simulink model "simulation1_eeef366_5"  (R2017a)
settings: Solver=ode1  StartTime=0.0  StopTime=24*3600  FixedStep=60  MaxStep=60  RelTol=1e-3  EnableMultiTasking=on
InitFcn:
  | clc
  | tic
  | disp('----------------------------------')
  | disp(' ### Solving...')
  | disp('----------------------------------')
StartFcn:
  | disp(['Initialization took: ', num2str(toc), ' s'])
  | disp('Solving...')
  | tic
StopFcn:
  | dt = str2double(get_param([gcs, '/', 'powergui'], 'SampleTime'));
  | 
  | tend = str2double(get_param(gcs, 'StopTime'));
  | 
  | runTime = toc;
  | disp('----------------------------------')
  | disp(['### Simulation took: ', num2str(runTime), ' secs'])
  | 
  | disp(['### Simulation took: ', num2str(runTime/60), ' mins'])
  | 
  | numSteps = tend / dt;
  | 
  | disp(['### Steps / sec = ', num2str(numSteps / runTime)])
  | 
  | disp(['### Secs / step = ', num2str(runTime / numSteps)])
  | 
  | disp(['### Num. steps = ', num2str(numSteps)])
  | disp('----------------------------------')
libraries: powerlib x60, powerlib_extras x12, powerlib_meascontrol x1
(part 1 of 2)
settings Model: Creator=fmu57  LastModifiedBy=Aryan Ritwajeet Jha
settings DataIOCC: LimitDataPoints=on  SaveFormat=Array  SignalLoggingSaveFormat=ModelDataLogs
settings OptimizationCC: ExpressionDepthLimit=2147483647  LifeSpan=inf
settings DebuggingCC: UnderspecifiedInitializationDetection=Classic  MergeDetectMultiDrivingBlocksExec=none  SolverPrmCheckMsg=warning  StateNameClashWarn=warning  SFUnexpectedBacktrackingDiag=warning  SFNoUnconditionalDefaultTransitionDiag=warning  SFExecutionAtInitializationDiag=none
settings HardwareCC: ProdBitPerPointer=32  ProdBitPerSizeT=32  ProdBitPerPtrDiffT=32  ProdLargestAtomicFloat=None  ProdIntDivRoundTo=Undefined  ProdEndianess=Unspecified  ProdWordSize=32  ProdHWDeviceType=32-bit Generic
settings ModelReferenceCC: PropagateSignalLabelsOutOfModel=off
settings GRTTargetCC: TargetLangStandard=C89/C90 (ANSI)  GeneratePreprocessorConditionals=Disable all  CombineOutputUpdateFcns=off  GRTInterface=on
settings ConfigComp: CovMetricSettings=dw  CovHtmlReporting=on  CovSaveCumulativeToWorkspaceVar=on  CovSaveSingleToWorkspaceVar=on  CovExternalEMLEnable=off

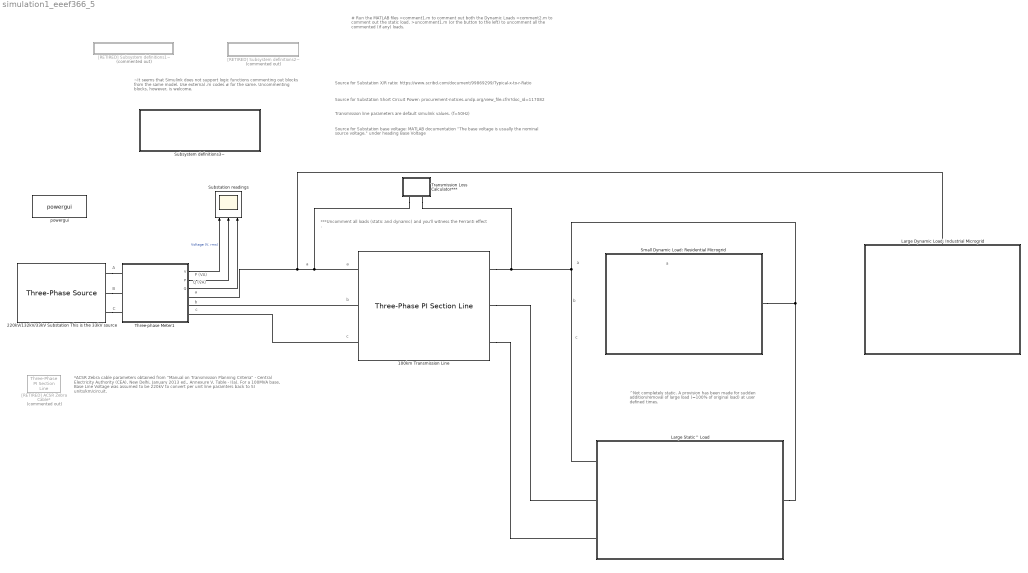
== system simulation1_eeef366_5 ==
  note: # Run the MATLAB files
      | >comment1.m to comment out both the Dynamic Loads
      | >comment2.m to comment out the static load.
      | >uncomment1.m (or the button to the left) to uncomment
      | all the commented (if any) loads.
  note: ~It seems that Simulink does not support
      | logic functions commenting out blocks
      | from the same model. Use external .m codes # for
      | the same. Uncommenting blocks, however, is welcome.
  note: ^Not completely static. A provision has
      | been made for sudden addition/removal of
      | large load (=100% of original load)
      | at user defined times.
  note: ***Uncomment all loads (static and dynamic) and you'll
      | witness the Ferranti effect .
  note: c
  note: b
  note: a
  note: a
  note: a
  note: c
  note: b
  note: a
  note: c
  note: b
  note: a
  note: C
  note: B
  note: A
  note: Q (VA)
  note: P (VA)
  note: Transmission line parameters are default simulink values. (f=50Hz)
  note: Source for Substation base voltage: MATLAB documentation "The base voltage is usually the nominal source voltage." under heading Base Voltage
  note: Source for Substation Short Circuit Power: procurement-notices.undp.org/view_file.cfm?doc_id=117082
  note: Source for Substation X/R ratio: https://www.scribd.com/document/99869299/Typical-x-to-r-Ratio
  note: *ACSR Zebra cable parameters obtained from
      | "Manual on Transmission Planning Criteria" - Central Electricity
      | Authority (CEA), New Delhi, January 2013 ed.,
      | Annexure V, Table - I(a). For a 100MVA base, Base Line Voltage was
      | assumed to be 220kV to convert per unit line paramters back
      | to SI units/km/circuit.
  " Subsystem definitions3~" : Subsystem
      settings: OpenFcn=uncomment1
      settings: CloseFcn=|
      | comment1
      | comment2
      mask Display: disp('Double Click me to Uncomment all loads')
  " [RETIRED] Subsystem definitions1~" : Subsystem  Commented=on
      settings: OpenFcn=comment1
      settings: CloseFcn=|
      | comment2
      | uncomment1
      mask Display: disp('Comment out Dynamic loads')
  " [RETIRED] Subsystem definitions2~" : Subsystem  Commented=on
      settings: OpenFcn=comment2
      settings: CloseFcn=|
      | comment1
      | uncomment1
      mask Display: disp('Comment out static loads')
  100km Transmission Line : powerlib/Elements/Three-Phase PI Section Line  LConnTagsString=a|b|c  RConnTagsString=A|B|C  Frequency=50  Resistances=[ 0.01273 0.3864]  Inductances="[ 0.9337e-3  4.1264e-3]"  Capacitances=[12.74e-9 7.751e-9]  Length=100  mask(Three-Phase PI Section Line){}
      settings: SourceProductName=Simscape Power Systems
      mask Display: image('C:\Users\Aryan Ritwajeet Jha\Desktop\CMS Desktop\3-2 2018-19\Mine\EEE F366\Foraged\Images\big-guard-500x500.jpg');
  220kV/132kV/33kV Substation This is the 33kV source : powerlib/Electrical Sources/Three-Phase Source  InternalConnection=Yg  VoltagePhases=off  Voltage=33e3  PhaseAngle=0  Voltage_phases=[25e3 25e3 25e3]/sqrt(3)  PhaseAngles_phases=[0 -120 +120]  Frequency=50  NonIdealSource=on  SpecifyImpedance=on  Resistance=1e-3  Inductance=1e-6  ShortCircuitLevel=sqrt(3)*33e3*25e3  BaseVoltage=33e3  XRratio=10  BusType=swing  Pref=0  Qref=0  Prefabc=[10e3, 10e3, 10e3]  Qrefabc=[0, 0, 0]  Qmin=-inf  Qmax=inf  mask(Three-Phase Source){}
      mask Display: image('C:\Users\Aryan Ritwajeet Jha\Desktop\CMS Desktop\3-2 2018-19\Mine\EEE F366\Foraged\Images\Substation.jpg');
  Large Dynamic Load: Industrial Microgrid : Subsystem
      mask Display: image('C:\Users\Aryan Ritwajeet Jha\Desktop\CMS Desktop\3-2 2018-19\Mine\EEE F366\Foraged\Images\landschaftspark_5.jpg');
  Large Static^ Load : Subsystem
      mask Display: image('C:\Users\Aryan Ritwajeet Jha\Desktop\CMS Desktop\3-2 2018-19\Mine\EEE F366\Foraged\Images\Chicagos-State-Street-corridor-public-housing-During-the-1960s-and-1970s-the-Chicago.png');
  Small Dynamic Load: Residential Microgrid : Subsystem
      mask Display: image('C:\Users\Aryan Ritwajeet Jha\Desktop\CMS Desktop\3-2 2018-19\Mine\EEE F366\Foraged\Images\central_garden_3_081214_tw630.jpg');
  Substation readings : Scope  NumInputPorts=3
  Three-phase Meter1 : Subsystem
      mask Display: image('C:\Users\Aryan Ritwajeet Jha\Desktop\CMS Desktop\3-2 2018-19\Mine\EEE F366\Foraged\Images\index4.jpg');
  Transmission Loss Calculator*** : Subsystem
  "[RETIRED] ACSR Zebra Cable* " : powerlib/Elements/Three-Phase PI Section Line  Commented=on  LConnTagsString=a|b|c  RConnTagsString=A|B|C  Frequency=50  Resistances=[ 0.00101 0.01858]  Inductances="[ 0.000067171  0.000242802]"  Capacitances=[0.119665371 0.197340289]  Length=16
      settings: SourceProductName=Simscape Power Systems
  powergui : powerlib/powergui  Priority=2  SimulationMode=Phasor  SampleTime=1  frequency=50  Iterations=50  frequencyindice=50  Pbase=100e6  ErrMax=1e-4  UnitsV=kV  UnitsW=MW  buscounter=0  FunctionMessages=off  echomessages=off  EnableUseOfTLC=off  CurrentSourceSwitches=off  DisableSnubberDevices=off  DisableRonSwitches=off  DisableVfSwitches=off  DisplayEquations=off  SolverType=Tustin  Interpol=off  ExternalGateDelay=off  methode=off  Ts=0  x0status=steady  SPID=off  SwTol=0  HookPort=off  RestoreLinks=warning  ResistiveCurrentMeasurement=off  Frange=logspace(0,3,50)  Ylog=off  Xlog=off  ShowGrid=off  save=off  variable=ZData  structure=0  ZoomFFT=on  StartTime=0.0  cycles=1  DisplayStyle=off  fundamental=60  FreqAxis=off  MaxFrequency=1000  frequencyindicesteady=1  RmsSteady=1  display=off
  wires:
  Three-phase Meter1/1(V) -> Substation readings/1  "Voltage (V, rms)"
  Three-phase Meter1/2(P) -> Substation readings/2
  Three-phase Meter1/3(Q) -> Substation readings/3
  connections:
  Transmission Loss Calculator***/LConn1 -- Large Dynamic Load: Industrial Microgrid/LConn1 -- Three-phase Meter1/RConn1 -- 100km Transmission Line/LConn1
  220kV/132kV/33kV Substation This is the 33kV source/RConn1 -- Three-phase Meter1/LConn1
  220kV/132kV/33kV Substation This is the 33kV source/RConn2 -- Three-phase Meter1/LConn2
  220kV/132kV/33kV Substation This is the 33kV source/RConn3 -- Three-phase Meter1/LConn3
  100km Transmission Line/LConn2 -- Three-phase Meter1/RConn2
  100km Transmission Line/LConn3 -- Three-phase Meter1/RConn3
  Transmission Loss Calculator***/LConn2 -- Large Static^ Load/RConn1 -- Small Dynamic Load: Residential Microgrid/LConn1 -- Large Static^ Load/LConn1 -- 100km Transmission Line/RConn1
  100km Transmission Line/RConn2 -- Large Static^ Load/LConn2
  100km Transmission Line/RConn3 -- Large Static^ Load/LConn3

== system simulation1_eeef366_5/ Subsystem definitions3~ ==

== system simulation1_eeef366_5/ [RETIRED] Subsystem definitions1~ ==

== system simulation1_eeef366_5/ [RETIRED] Subsystem definitions2~ ==

== system simulation1_eeef366_5/Large Dynamic Load: Industrial Microgrid ==
  note: **Image of an actual industrial complex embedded in a solar farm in China
  Center tapped Industrial T/F 1 50MVA 33kV(LL)/240V/240V : powerlib/Elements/Linear Transformer  Tag=tf1  UNITS=SI  NominalPower=[50e6,50]  winding1=[33e3/sqrt(3) 0 0]  winding2=[240 0 0]  ThreeWindings=on  winding3=[240 0 0]  RmLm=[1e6 inf]  Measurements=None  DataType=on
  Ground3 : powerlib/Elements/Ground  LConnTagsString=a
  Ground4 : powerlib/Elements/Ground  LConnTagsString=a
  Ground5 : powerlib/Elements/Ground  LConnTagsString=a
  Industrial Area Smart Meter : Subsystem
      mask Display: image('C:\Users\Aryan Ritwajeet Jha\Desktop\CMS Desktop\3-2 2018-19\Mine\EEE F366\Foraged\Images\1115.png');
  Smart Industrial Complex** : Subsystem
      mask Display: image('C:\Users\Aryan Ritwajeet Jha\Desktop\CMS Desktop\3-2 2018-19\Mine\EEE F366\Foraged\Images\p06j7zyr.jpg');
  Total Smart Industrial Area Readings : Scope  NumInputPorts=5
  Conn1 : PMIOPort  Port=1  Side=Left
  wires:
  Smart Industrial Complex**/3(Out3) -> Total Smart Industrial Area Readings/4
  Smart Industrial Complex**/1(Out1) -> Total Smart Industrial Area Readings/2
  Smart Industrial Complex**/2(Out2) -> Total Smart Industrial Area Readings/3
  Industrial Area Smart Meter/1(V) -> Total Smart Industrial Area Readings/1  "Voltage (V, rms)"
  Industrial Area Smart Meter/2(P,Q) -> Total Smart Industrial Area Readings/5
  connections:
  Center tapped Industrial T/F 1 50MVA 33kV(LL)/240V/240V/LConn1 -- Conn1/RConn1
  Center tapped Industrial T/F 1 50MVA 33kV(LL)/240V/240V/RConn4 -- Industrial Area Smart Meter/LConn3
  Center tapped Industrial T/F 1 50MVA 33kV(LL)/240V/240V/LConn2 -- Ground5/LConn1
  Industrial Area Smart Meter/RConn2 -- Smart Industrial Complex**/LConn2
  Ground4/LConn1 -- Industrial Area Smart Meter/LConn2
  Industrial Area Smart Meter/RConn1 -- Smart Industrial Complex**/LConn1
  Industrial Area Smart Meter/RConn3 -- Smart Industrial Complex**/LConn3
  Center tapped Industrial T/F 1 50MVA 33kV(LL)/240V/240V/RConn2 -- Ground3/LConn1 -- Center tapped Industrial T/F 1 50MVA 33kV(LL)/240V/240V/RConn3
  Center tapped Industrial T/F 1 50MVA 33kV(LL)/240V/240V/RConn1 -- Industrial Area Smart Meter/LConn1

== system simulation1_eeef366_5/Large Static^ Load ==
  note: [10AM to 01PM]
      | [08PM to 10PM]
  Extra (Peak) Load [1MW + j0.2MW] : powerlib/Elements/Three-Phase Series RLC Load  LConnTagsString=A|B|C  Configuration=Y (grounded)  NominalVoltage=[33e3]  Vabc=[1e3 1e3 1e3]  Vabcp=[1e3 1e3 1e3]  NominalFrequency=50  UnbalancedPower=off  ActivePower=1e6  InductivePower=2e5  CapacitivePower=0  Pabc=[10e3 9e3 11e3]  QLabc=[100 90 110]  QCabc=[100 90 110]  Pabcp=[10e3 9e3 11e3]  QLabcp=[100 90 110]  QCabcp=[100 90 110]  Measurements=None  LoadType=constant Z  mask(Three-Phase Series RLC Load){}
      mask Display: image('C:\Users\Aryan Ritwajeet Jha\Desktop\CMS Desktop\3-2 2018-19\Mine\EEE F366\Foraged\Images\Purple-Dallas-skyline.jpg');
  Permanent Load [1MW + j0.2MW] : powerlib/Elements/Three-Phase Series RLC Load  LConnTagsString=A|B|C  Configuration=Y (grounded)  NominalVoltage=[33e3]  Vabc=[1e3 1e3 1e3]  Vabcp=[1e3 1e3 1e3]  NominalFrequency=50  UnbalancedPower=off  ActivePower=1e6  InductivePower=2e5  CapacitivePower=0  Pabc=[10e3 9e3 11e3]  QLabc=[100 90 110]  QCabc=[100 90 110]  Pabcp=[10e3 9e3 11e3]  QLabcp=[100 90 110]  QCabcp=[100 90 110]  Measurements=None  LoadType=constant Z  mask(Three-Phase Series RLC Load){}
      mask Display: image('C:\Users\Aryan Ritwajeet Jha\Desktop\CMS Desktop\3-2 2018-19\Mine\EEE F366\Foraged\Images\new_york_city_skyline_looking-1600x900.jpg');
  Three-Phase Breaker : powerlib/Elements/Three-Phase Breaker  InitialState=open  SwitchA=on  SwitchB=on  SwitchC=on  SwitchTimes=[10*3600 46800 72000 79200]  External=off  BreakerResistance=0.01  SnubberResistance=1e6  SnubberCapacitance=inf  Measurements=None  mask(Three-Phase Breaker){}
      mask Display: image('C:\Users\Aryan Ritwajeet Jha\Desktop\CMS Desktop\3-2 2018-19\Mine\EEE F366\Foraged\Images\41bXoEJnQnL.jpg');
  Conn1 : PMIOPort  Port=1  Side=Left
  Conn2 : PMIOPort  Port=2  Side=Right
  Conn3 : PMIOPort  Port=3  Side=Left
  Conn4 : PMIOPort  Port=4  Side=Left
  connections:
  Permanent Load [1MW + j0.2MW]/LConn1 -- Conn1/RConn1
  Three-Phase Breaker/RConn1 -- Conn2/RConn1
  Extra (Peak) Load [1MW + j0.2MW]/LConn1 -- Three-Phase Breaker/LConn1
  Extra (Peak) Load [1MW + j0.2MW]/LConn2 -- Three-Phase Breaker/LConn2
  Permanent Load [1MW + j0.2MW]/LConn2 -- Conn3/RConn1 -- Three-Phase Breaker/RConn2
  Extra (Peak) Load [1MW + j0.2MW]/LConn3 -- Three-Phase Breaker/LConn3
  Three-Phase Breaker/RConn3 -- Conn4/RConn1 -- Permanent Load [1MW + j0.2MW]/LConn3

== system simulation1_eeef366_5/Small Dynamic Load: Residential Microgrid ==
  Center tapped Residential T/F 2 2500kVA 33kV(LL)/120V/120V : powerlib/Elements/Linear Transformer  UNITS=SI  NominalPower=[2500e3,50]  winding1=[33e3/sqrt(3) 0 0]  winding2=[120 0 0]  ThreeWindings=on  winding3=[120 0 0]  RmLm=[1e6 inf]  Measurements=None  DataType=on
  Ground1 : powerlib/Elements/Ground  LConnTagsString=a
  Ground2 : powerlib/Elements/Ground  LConnTagsString=a
  Ground6 : powerlib/Elements/Ground  LConnTagsString=a
  Residential Area Smart Meter : Subsystem
      mask Display: image('C:\Users\Aryan Ritwajeet Jha\Desktop\CMS Desktop\3-2 2018-19\Mine\EEE F366\Foraged\Images\1115.png');
  Smart Residential Complex : Subsystem
      mask Display: image('C:\Users\Aryan Ritwajeet Jha\Desktop\CMS Desktop\3-2 2018-19\Mine\EEE F366\Foraged\Images\energy-efficiency.jpg');
  Total Smart Residential Area Readings : Scope  NumInputPorts=5
  Conn1 : PMIOPort  Port=1  Side=Left
  wires:
  Residential Area Smart Meter/1(V) -> Total Smart Residential Area Readings/1  "Voltage (V, rms)"
  Smart Residential Complex/3(Out3) -> Total Smart Residential Area Readings/4
  Smart Residential Complex/2(Out2) -> Total Smart Residential Area Readings/3
  Smart Residential Complex/1(Out1) -> Total Smart Residential Area Readings/2
  Residential Area Smart Meter/2(P,Q) -> Total Smart Residential Area Readings/5  "Power (W, Vars)"
  connections:
  Center tapped Residential T/F 2 2500kVA 33kV(LL)/120V/120V/LConn1 -- Conn1/RConn1
  Center tapped Residential T/F 2 2500kVA 33kV(LL)/120V/120V/LConn2 -- Ground6/LConn1
  Residential Area Smart Meter/RConn3 -- Smart Residential Complex/LConn3
  Center tapped Residential T/F 2 2500kVA 33kV(LL)/120V/120V/RConn4 -- Residential Area Smart Meter/LConn3
  Center tapped Residential T/F 2 2500kVA 33kV(LL)/120V/120V/RConn1 -- Residential Area Smart Meter/LConn1
  Center tapped Residential T/F 2 2500kVA 33kV(LL)/120V/120V/RConn2 -- Ground1/LConn1 -- Center tapped Residential T/F 2 2500kVA 33kV(LL)/120V/120V/RConn3
  Residential Area Smart Meter/RConn1 -- Smart Residential Complex/LConn1
  Residential Area Smart Meter/RConn2 -- Smart Residential Complex/LConn2
  Ground2/LConn1 -- Residential Area Smart Meter/LConn2

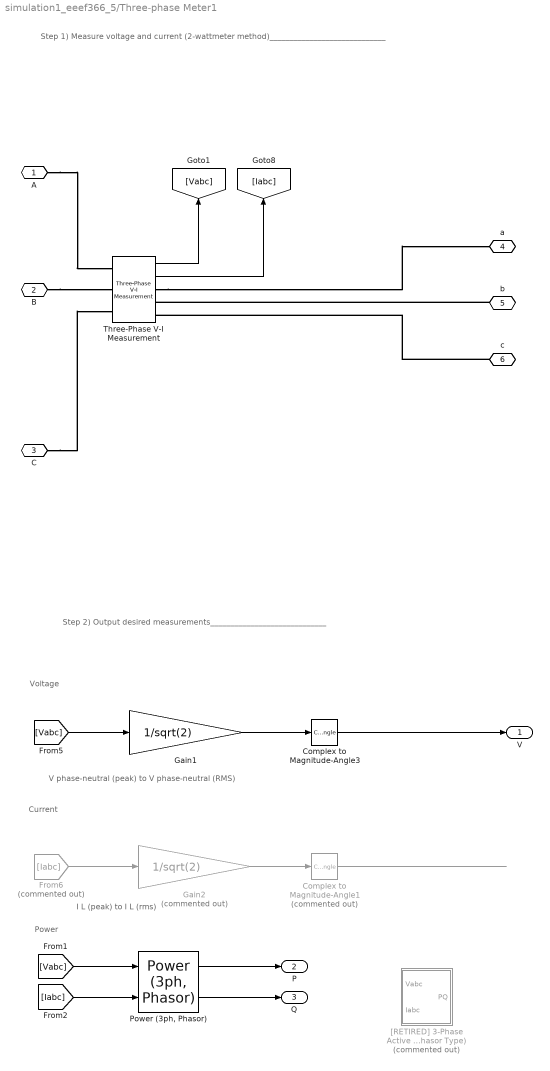
== system simulation1_eeef366_5/Three-phase Meter1 ==
  note: Step 1) Measure voltage and current (2-wattmeter method)_____________________________
  note: Step 2) Output desired measurements_____________________________
  note: Power
  note: Current
  note: Voltage
  note: V phase-neutral (peak) to V phase-neutral (RMS)
  note: I L (peak) to I L (rms)
  Complex to Magnitude-Angle1 : ComplexToMagnitudeAngle  Commented=on  Output=Magnitude
  Complex to Magnitude-Angle3 : ComplexToMagnitudeAngle  Output=Magnitude
  From6 : From  Commented=on  GotoTag=Iabc
  Gain1 : Gain  Gain=1/sqrt(2)
  Gain2 : Gain  Commented=on  Gain=1/sqrt(2)
  "Power (3ph, Phasor)" : powerlib_meascontrol/Measurements/Power (3ph, Phasor)
      settings: SourceProductName=Simscape Power Systems  SourceProductBaseCode=PS
  Three-Phase V-I Measurement : powerlib/Measurements/Three-Phase V-I Measurement  VoltageMeasurement=phase-to-ground  SetLabelV=off  LabelV=Vabc  Vpu=off  VpuLL=off  CurrentMeasurement=yes  SetLabelI=off  LabelI=Iabc  Ipu=off  Pbase=100e6  Vbase=500e3  OutputType=Complex  PhasorSimulation=on  PSBequivalent=0
  "[RETIRED] 3-Phase Active & Reactive Power (Phasor Type)" : Subsystem  Commented=on  AncestorBlock=|  DialogController=POWERSYS.PowerSysDialog  mask(3-Phase Active & Reactive Power (Phasor Type)){}
      | powerlib_extras/Phasor
      | Library/3-Phase
      | Active & Reactive Power
      | (Phasor Type)
      mask help: 3-Phase Active & Reactive Power (Phasor Type)
      mask init:
      | power_initmask();
      mask Help: This block is part of a subset of blocks in the Extras library that does not have documentation associated with it, other than the block mask description.
      mask Display: disp('')
  A : PMIOPort  Port=1  Side=Left
      settings: AttributesFormatString=%<Side>
  B : PMIOPort  Port=2  Side=Left
      settings: AttributesFormatString=%<Side>
  C : PMIOPort  Port=3  Side=Left
      settings: AttributesFormatString=%<Side>
  a : PMIOPort  Port=4  Side=Right
      settings: AttributesFormatString=%<Side>
  b : PMIOPort  Port=5  Side=Right
      settings: AttributesFormatString=%<Side>
  c : PMIOPort  Port=6  Side=Right
      settings: AttributesFormatString=%<Side>
  V : Outport
  P : Outport  Port=2
  Q : Outport  Port=3
  wires:
  Gain1/1 -> Complex to Magnitude-Angle3/1
  Complex to Magnitude-Angle3/1 -> V/1
  [Vabc] -> Gain1/1
  Gain2/1 -> Complex to Magnitude-Angle1/1
  Complex to Magnitude-Angle1/1 -> ?
  From6/1 -> Gain2/1
  Three-Phase V-I Measurement/2 -> [Iabc]
  Three-Phase V-I Measurement/1 -> [Vabc]
  "Power (3ph, Phasor)"/1 -> P/1
  "Power (3ph, Phasor)"/2 -> Q/1
  [Vabc] -> "Power (3ph, Phasor)"/1
  [Iabc] -> "Power (3ph, Phasor)"/2
  connections:
  A/RConn1 -- Three-Phase V-I Measurement/LConn1
  B/RConn1 -- Three-Phase V-I Measurement/LConn2
  C/RConn1 -- Three-Phase V-I Measurement/LConn3
  Three-Phase V-I Measurement/RConn1 -- a/RConn1
  b/RConn1 -- Three-Phase V-I Measurement/RConn2
  c/RConn1 -- Three-Phase V-I Measurement/RConn3

== system simulation1_eeef366_5/Transmission Loss Calculator*** ==
  note: Subsystem2
  note: Subsystem1
  Complex to Magnitude-Angle : ComplexToMagnitudeAngle  Output=Magnitude
  Complex to Magnitude-Angle1 : ComplexToMagnitudeAngle  Output=Magnitude
  Gain : Gain  Gain=1/sqrt(2)
  Gain1 : Gain  Gain=1/sqrt(2)
  Ground1 : powerlib/Elements/Ground  LConnTagsString=a
  Ground7 : powerlib/Elements/Ground  LConnTagsString=a
  Receiving Voltage : Display
  Sending Voltage : Display
  Voltage Measurement : powerlib/Measurements/Voltage Measurement  PhasorSimulation=on  OutputType=Complex  PSBequivalent=0
  Voltage Measurement1 : powerlib/Measurements/Voltage Measurement  PhasorSimulation=on  OutputType=Complex  PSBequivalent=0
  Vs : PMIOPort  Port=1  Side=Left
  Vr : PMIOPort  Port=2  Side=Left
  wires:
  Complex to Magnitude-Angle/1 -> Gain/1
  Voltage Measurement/1 -> Complex to Magnitude-Angle/1
  Complex to Magnitude-Angle1/1 -> Gain1/1
  Voltage Measurement1/1 -> Complex to Magnitude-Angle1/1
  Gain1/1 -> Sending Voltage/1
  Gain/1 -> Receiving Voltage/1
  connections:
  Voltage Measurement1/LConn1 -- Vs/RConn1
  Voltage Measurement/LConn1 -- Vr/RConn1
  Ground7/LConn1 -- Voltage Measurement/LConn2
  Ground1/LConn1 -- Voltage Measurement1/LConn2

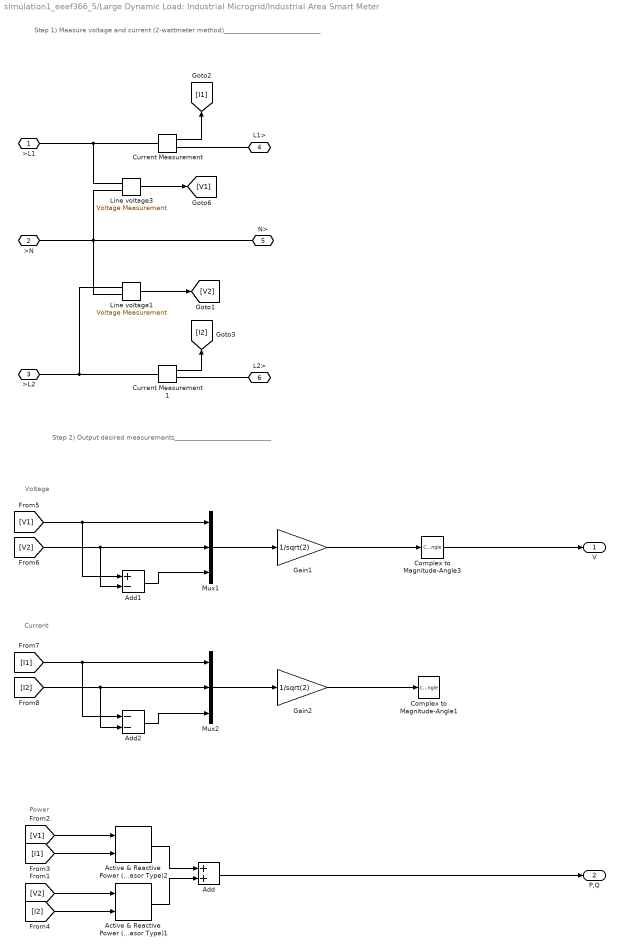
== system simulation1_eeef366_5/Large Dynamic Load: Industrial Microgrid/Industrial Area Smart Meter ==
  note: Voltage
  note: Current
  note: Power
  note: Step 2) Output desired measurements_____________________________
  note: Step 1) Measure voltage and current (2-wattmeter method)_____________________________
  Active & Reactive Power (Phasor Type)1 : powerlib_extras/Phasor Library/Active & Reactive Power (Phasor Type)
  Active & Reactive Power (Phasor Type)2 : powerlib_extras/Phasor Library/Active & Reactive Power (Phasor Type)
  Add : Sum
  Add1 : Sum  Inputs=+-
  Add2 : Sum  Inputs=--
  Complex to Magnitude-Angle1 : ComplexToMagnitudeAngle  Output=Magnitude
  Complex to Magnitude-Angle3 : ComplexToMagnitudeAngle  Output=Magnitude
  Current Measurement : powerlib/Measurements/Current Measurement  PhasorSimulation=on  OutputType=Complex  PSBequivalent=0
  Current Measurement1 : powerlib/Measurements/Current Measurement  PhasorSimulation=on  OutputType=Complex  PSBequivalent=0
  Gain1 : Gain  Gain=1/sqrt(2)
  Gain2 : Gain  Gain=1/sqrt(2)
  Line voltage1 : powerlib/Measurements/Voltage Measurement  Tag=PoWeRsYsTeMmEaSuReMeNt  PhasorSimulation=on  OutputType=Complex  PSBequivalent=0
  Line voltage3 : powerlib/Measurements/Voltage Measurement  Tag=PoWeRsYsTeMmEaSuReMeNt  PhasorSimulation=on  OutputType=Complex  PSBequivalent=0
  Mux1 : Mux  Inputs=3
  Mux2 : Mux  Inputs=3
  >L1 : PMIOPort  Port=1  Side=Left
      settings: AttributesFormatString=%<Side>
  >N : PMIOPort  Port=2  Side=Left
      settings: AttributesFormatString=%<Side>
  >L2 : PMIOPort  Port=3  Side=Left
      settings: AttributesFormatString=%<Side>
  L1> : PMIOPort  Port=4  Side=Right
      settings: AttributesFormatString=%<Side>
  N> : PMIOPort  Port=5  Side=Right
      settings: AttributesFormatString=%<Side>
  L2> : PMIOPort  Port=6  Side=Right
      settings: AttributesFormatString=%<Side>
  V : Outport
  P,Q : Outport  Port=2
  wires:
  Complex to Magnitude-Angle3/1 -> V/1
  Gain2/1 -> Complex to Magnitude-Angle1/1
  Gain1/1 -> Complex to Magnitude-Angle3/1
  Mux2/1 -> Gain2/1
  Add2/1 -> Mux2/3
  [I2] -> Mux2/2, Add2/2
  [I1] -> Mux2/1, Add2/1
  Mux1/1 -> Gain1/1
  Add1/1 -> Mux1/3
  [V2] -> Add1/2, Mux1/2
  [V1] -> Add1/1, Mux1/1
  Add/1 -> P,Q/1
  Active & Reactive Power (Phasor Type)1/1 -> Add/2
  Active & Reactive Power (Phasor Type)2/1 -> Add/1
  [I2] -> Active & Reactive Power (Phasor Type)1/2
  [V2] -> Active & Reactive Power (Phasor Type)1/1
  [I1] -> Active & Reactive Power (Phasor Type)2/2
  [V1] -> Active & Reactive Power (Phasor Type)2/1
  Current Measurement1/1 -> [I2]
  Current Measurement/1 -> [I1]
  Line voltage1/1 -> [V2]
  Line voltage3/1 -> [V1]
  connections:
  L2>/RConn1 -- Current Measurement1/RConn1
  Current Measurement1/LConn1 -- Line voltage1/LConn1 -- >L2/RConn1
  >N/RConn1 -- Line voltage1/LConn2 -- Line voltage3/LConn2 -- N>/RConn1
  Current Measurement/RConn1 -- L1>/RConn1
  Line voltage3/LConn1 -- Current Measurement/LConn1 -- >L1/RConn1

== system simulation1_eeef366_5/Large Dynamic Load: Industrial Microgrid/Smart Industrial Complex** ==
  Add : Sum
  Add1 : Sum
  Add2 : Sum
  Distributed Generators for Industry01 (Customized Profile) : Subsystem
      mask Display: image('C:\Users\Aryan Ritwajeet Jha\Pictures\Icons8 added\icons8_Greentech_64.png');
  Distributed Generators for Industry02 (Customized Profile) : Subsystem
      mask Display: image('C:\Users\Aryan Ritwajeet Jha\Pictures\Icons8 added\icons8_Greentech_64.png');
  Industry01 : Subsystem  AncestorBlock=libraryMyTools/homeGroupData1
      mask Display: image('C:\Users\Aryan Ritwajeet Jha\Desktop\CMS Desktop\3-2 2018-19\Mine\EEE F366\Foraged\Images\p06j7zyr.jpg');
  Industry01 Readings : Scope  NumInputPorts=5
  Industry02 : Subsystem  AncestorBlock=libraryMyTools/homeGroupData1
      mask Display: image('C:\Users\Aryan Ritwajeet Jha\Desktop\CMS Desktop\3-2 2018-19\Mine\EEE F366\Foraged\Images\p06j7zyr.jpg');
  Industry02 Readings : Scope  NumInputPorts=5
  Smart Meter Industry01 : Subsystem
      mask Display: image('C:\Users\Aryan Ritwajeet Jha\Desktop\CMS Desktop\3-2 2018-19\Mine\EEE F366\Foraged\Images\1115.png');
  Smart Meter Industry02 : Subsystem
      mask Display: image('C:\Users\Aryan Ritwajeet Jha\Desktop\CMS Desktop\3-2 2018-19\Mine\EEE F366\Foraged\Images\1115.png');
  L1 : PMIOPort  Tag=PMCPort  Port=1  Side=Left
  N : PMIOPort  Tag=PMCPort  Port=2  Side=Left
  L2 : PMIOPort  Tag=PMCPort  Port=3  Side=Left
  Out1 : Outport
  Out2 : Outport  Port=2
  Out3 : Outport  Port=3
  wires:
  Distributed Generators for Industry01 (Customized Profile)/3(Out3) -> Add2/2, Industry01 Readings/4
  Distributed Generators for Industry01 (Customized Profile)/2(Out2) -> Add1/1, Industry01 Readings/3
  Smart Meter Industry01/3(P,Q) -> Industry01 Readings/5  "Power (W)"
  Smart Meter Industry01/1(V) -> Industry01 Readings/1  "Voltage (V, rms)"
  Distributed Generators for Industry01 (Customized Profile)/1(Out1) -> Add/1, Industry01 Readings/2
  Distributed Generators for Industry01 (Customized Profile)/4(Out4) -> Industry01/1(Total Industry01 power consumption.csv (VA))
  Smart Meter Industry02/1(V) -> Industry02 Readings/1  "Voltage (V, rms)"
  Smart Meter Industry02/3(P,Q) -> Industry02 Readings/5  "Power (W)"
  Distributed Generators for Industry02 (Customized Profile)/3(Out3) -> Add2/1, Industry02 Readings/4
  Distributed Generators for Industry02 (Customized Profile)/4(Out4) -> Industry02/1(Total Industry02 power consumption.csv (VA))
  Distributed Generators for Industry02 (Customized Profile)/2(Out2) -> Add1/2, Industry02 Readings/3
  Add/1 -> Out1/1
  Add2/1 -> Out3/1
  Add1/1 -> Out2/1
  Distributed Generators for Industry02 (Customized Profile)/1(Out1) -> Add/2, Industry02 Readings/2
  connections:
  Industry02/LConn1 -- Smart Meter Industry02/RConn1
  Industry02/LConn2 -- Smart Meter Industry02/RConn2
  Industry02/LConn3 -- Smart Meter Industry02/RConn3
  Industry01/LConn1 -- Smart Meter Industry01/RConn1
  Industry01/LConn2 -- Smart Meter Industry01/RConn2
  Industry01/LConn3 -- Smart Meter Industry01/RConn3
  Smart Meter Industry02/LConn1 -- L1/RConn1 -- Smart Meter Industry01/LConn1
  Smart Meter Industry02/LConn2 -- N/RConn1 -- Smart Meter Industry01/LConn2
  Smart Meter Industry02/LConn3 -- L2/RConn1 -- Smart Meter Industry01/LConn3

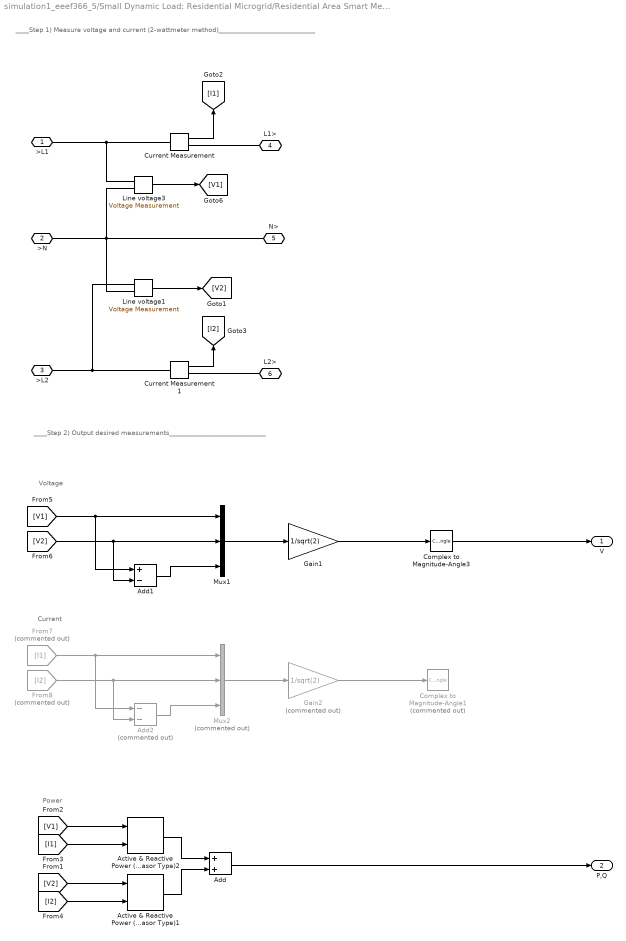
== system simulation1_eeef366_5/Small Dynamic Load: Residential Microgrid/Residential Area Smart Meter ==
  note: Voltage
  note: Current
  note: Power
  note: ____Step 2) Output desired measurements_____________________________
  note: ____Step 1) Measure voltage and current (2-wattmeter method)_____________________________
  Active & Reactive Power (Phasor Type)1 : powerlib_extras/Phasor Library/Active & Reactive Power (Phasor Type)
  Active & Reactive Power (Phasor Type)2 : powerlib_extras/Phasor Library/Active & Reactive Power (Phasor Type)
  Add : Sum
  Add1 : Sum  Inputs=+-
  Add2 : Sum  Commented=on  Inputs=--
  Complex to Magnitude-Angle1 : ComplexToMagnitudeAngle  Commented=on  Output=Magnitude
  Complex to Magnitude-Angle3 : ComplexToMagnitudeAngle  Output=Magnitude
  Current Measurement : powerlib/Measurements/Current Measurement  PhasorSimulation=on  OutputType=Complex  PSBequivalent=0
  Current Measurement1 : powerlib/Measurements/Current Measurement  PhasorSimulation=on  OutputType=Complex  PSBequivalent=0
  From7 : From  Commented=on  GotoTag=I1
  From8 : From  Commented=on  GotoTag=I2
  Gain1 : Gain  Gain=1/sqrt(2)
  Gain2 : Gain  Commented=on  Gain=1/sqrt(2)
  Line voltage1 : powerlib/Measurements/Voltage Measurement  Tag=PoWeRsYsTeMmEaSuReMeNt  PhasorSimulation=on  OutputType=Complex  PSBequivalent=0
  Line voltage3 : powerlib/Measurements/Voltage Measurement  Tag=PoWeRsYsTeMmEaSuReMeNt  PhasorSimulation=on  OutputType=Complex  PSBequivalent=0
  Mux1 : Mux  Inputs=3
  Mux2 : Mux  Commented=on  Inputs=3
  >L1 : PMIOPort  Port=1  Side=Left
      settings: AttributesFormatString=%<Side>
  >N : PMIOPort  Port=2  Side=Left
      settings: AttributesFormatString=%<Side>
  >L2 : PMIOPort  Port=3  Side=Left
      settings: AttributesFormatString=%<Side>
  L1> : PMIOPort  Port=4  Side=Right
      settings: AttributesFormatString=%<Side>
  N> : PMIOPort  Port=5  Side=Right
      settings: AttributesFormatString=%<Side>
  L2> : PMIOPort  Port=6  Side=Right
      settings: AttributesFormatString=%<Side>
  V : Outport
  P,Q : Outport  Port=2
  wires:
  Complex to Magnitude-Angle3/1 -> V/1
  Gain2/1 -> Complex to Magnitude-Angle1/1
  Gain1/1 -> Complex to Magnitude-Angle3/1
  Mux2/1 -> Gain2/1
  Add2/1 -> Mux2/3
  From8/1 -> Mux2/2, Add2/2
  From7/1 -> Mux2/1, Add2/1
  Mux1/1 -> Gain1/1
  Add1/1 -> Mux1/3
  [V2] -> Add1/2, Mux1/2
  [V1] -> Add1/1, Mux1/1
  Add/1 -> P,Q/1
  Active & Reactive Power (Phasor Type)1/1 -> Add/2
  Active & Reactive Power (Phasor Type)2/1 -> Add/1
  [I2] -> Active & Reactive Power (Phasor Type)1/2
  [V2] -> Active & Reactive Power (Phasor Type)1/1
  [I1] -> Active & Reactive Power (Phasor Type)2/2
  [V1] -> Active & Reactive Power (Phasor Type)2/1
  Current Measurement1/1 -> [I2]
  Current Measurement/1 -> [I1]
  Line voltage1/1 -> [V2]
  Line voltage3/1 -> [V1]
  connections:
  L2>/RConn1 -- Current Measurement1/RConn1
  Current Measurement1/LConn1 -- Line voltage1/LConn1 -- >L2/RConn1
  >N/RConn1 -- Line voltage1/LConn2 -- Line voltage3/LConn2 -- N>/RConn1
  Current Measurement/RConn1 -- L1>/RConn1
  Line voltage3/LConn1 -- Current Measurement/LConn1 -- >L1/RConn1

== system simulation1_eeef366_5/Small Dynamic Load: Residential Microgrid/Smart Residential Complex ==
  Add : Sum
  Add1 : Sum
  Add2 : Sum
  Distributed Generators for House01 : Subsystem
      mask Display: image('C:\Users\Aryan Ritwajeet Jha\Pictures\Icons8 added\icons8_Greentech_64.png');
  Distributed Generators for House2 : Subsystem
      mask Display: image('C:\Users\Aryan Ritwajeet Jha\Pictures\Icons8 added\icons8_Greentech_64.png');
  House01 Readings : Scope  NumInputPorts=5
  House02 Readings : Scope  NumInputPorts=5
  House1 : Subsystem  AncestorBlock=libraryMyTools/homeGroupData1
      mask Display: image('C:\Users\Aryan Ritwajeet Jha\Desktop\CMS Desktop\3-2 2018-19\Mine\EEE F366\Foraged\Images\energy-efficiency.jpg');
  House2 : Subsystem  AncestorBlock=libraryMyTools/homeGroupData1
      mask Display: image('C:\Users\Aryan Ritwajeet Jha\Desktop\CMS Desktop\3-2 2018-19\Mine\EEE F366\Foraged\Images\energy-efficiency.jpg');
  Smart Meter House01 : Subsystem
      mask Display: image('C:\Users\Aryan Ritwajeet Jha\Desktop\CMS Desktop\3-2 2018-19\Mine\EEE F366\Foraged\Images\1115.png');
  Smart Meter House02 : Subsystem
      mask Display: image('C:\Users\Aryan Ritwajeet Jha\Desktop\CMS Desktop\3-2 2018-19\Mine\EEE F366\Foraged\Images\1115.png');
  L1 : PMIOPort  Tag=PMCPort  Port=1  Side=Left
  N : PMIOPort  Tag=PMCPort  Port=2  Side=Left
  L2 : PMIOPort  Tag=PMCPort  Port=3  Side=Left
  Out1 : Outport
  Out2 : Outport  Port=2
  Out3 : Outport  Port=3
  wires:
  Smart Meter House01/1(V) -> House01 Readings/1  "Voltage (V, rms)"
  Smart Meter House01/3(P,Q) -> House01 Readings/5  "Power (W)"
  Distributed Generators for House01/1(Out1) -> Add/1, House01 Readings/2
  Distributed Generators for House01/2(Out2) -> Add1/1, House01 Readings/3
  Distributed Generators for House01/3(Out3) -> Add2/1, House01 Readings/4
  Distributed Generators for House01/4(Out4) -> House1/1(Total House01 power consumption.csv (VA))
  Distributed Generators for House2/3(Out3) -> Add2/2, House02 Readings/4
  Distributed Generators for House2/2(Out2) -> Add1/2, House02 Readings/3
  Smart Meter House02/3(P,Q) -> House02 Readings/5  "Power (W)"
  Smart Meter House02/1(V) -> House02 Readings/1  "Voltage (V, rms)"
  Distributed Generators for House2/1(Out1) -> Add/2, House02 Readings/2
  Distributed Generators for House2/4(Out4) -> House2/1(Total House02 power consumption.csv (VA))
  Add/1 -> Out1/1
  Add1/1 -> Out2/1
  Add2/1 -> Out3/1
  connections:
  House2/LConn1 -- Smart Meter House02/RConn1
  House2/LConn2 -- Smart Meter House02/RConn2
  House2/LConn3 -- Smart Meter House02/RConn3
  House1/LConn1 -- Smart Meter House01/RConn1
  House1/LConn2 -- Smart Meter House01/RConn2
  House1/LConn3 -- Smart Meter House01/RConn3
  Smart Meter House02/LConn1 -- L1/RConn1 -- Smart Meter House01/LConn1
  Smart Meter House02/LConn2 -- N/RConn1 -- Smart Meter House01/LConn2
  Smart Meter House02/LConn3 -- L2/RConn1 -- Smart Meter House01/LConn3

== system simulation1_eeef366_5/Three-phase Meter1/[RETIRED] 3-Phase Active & Reactive Power (Phasor Type) ==
  Vabc : Inport  PortDimensions=3
  Iabc : Inport  Port=2  PortDimensions=3
  Complex to Real-Imag : ComplexToRealImag
  K : Gain  Gain=1/2  SaturateOnIntegerOverflow=on  OutDataTypeStr=Inherit: Same as input  ParamDataTypeStr=Inherit: Same as input
  Math Function : Math  Operator=conj  SaturateOnIntegerOverflow=on
  Mux : Mux  Inputs=2
  Product2 : Product  SaturateOnIntegerOverflow=on  InputSameDT=on  OutDataTypeStr=Inherit: Same as first input
  Sum3 : Sum  Inputs=1  SaturateOnIntegerOverflow=on  InputSameDT=on  OutDataTypeStr=Inherit: Same as first input
  PQ : Outport
  wires:
  Mux/1 -> PQ/1
  Complex to Real-Imag/2 -> Mux/2
  Complex to Real-Imag/1 -> Mux/1
  K/1 -> Complex to Real-Imag/1
  Sum3/1 -> K/1
  Product2/1 -> Sum3/1
  Math Function/1 -> Product2/2
  Vabc/1 -> Product2/1
  Iabc/1 -> Math Function/1

== system simulation1_eeef366_5/Large Dynamic Load: Industrial Microgrid/Smart Industrial Complex**/Distributed Generators for Industry01 (Customized Profile) ==
  Gain{1..3,5} (4 alike) : Gain  Gain=1e6
  Industry01 Power Consumption : FromWorkspace  VariableName=industryphouse01  OutputAfterFinalValue=Holding final value
      mask Display: image('C:\Users\Aryan Ritwajeet Jha\Desktop\CMS Desktop\3-2 2018-19\Mine\EEE F366\Foraged\Images\images.jpg');
  Power transaction with Electric Utility : FromWorkspace  VariableName=industry01  OutputAfterFinalValue=Holding final value
      mask Display: image('C:\Users\Aryan Ritwajeet Jha\Desktop\CMS Desktop\3-2 2018-19\Mine\EEE F366\Foraged\Images\index3.jpg');
  Solar Power : FromWorkspace  VariableName=industrypsolar01  OutputAfterFinalValue=Holding final value
      mask Display: image('C:\Users\Aryan Ritwajeet Jha\Desktop\CMS Desktop\3-2 2018-19\Mine\EEE F366\Foraged\Images\MIT-PPA-1_0.jpg');
  Wind Power : FromWorkspace  VariableName=industrypwind01  OutputAfterFinalValue=Holding final value
      mask Display: image('C:\Users\Aryan Ritwajeet Jha\Desktop\CMS Desktop\3-2 2018-19\Mine\EEE F366\Foraged\Images\index2.jpg');
  Out1 : Outport
  Out2 : Outport  Port=2
  Out3 : Outport  Port=3
  Out4 : Outport  Port=4
  wires:
  Gain3/1 -> Out4/1
  Power transaction with Electric Utility/1 -> Gain3/1
  Wind Power/1 -> Gain2/1
  Solar Power/1 -> Gain1/1
  Gain5/1 -> Out1/1
  Industry01 Power Consumption/1 -> Gain5/1
  Gain1/1 -> Out2/1
  Gain2/1 -> Out3/1

== system simulation1_eeef366_5/Large Dynamic Load: Industrial Microgrid/Smart Industrial Complex**/Distributed Generators for Industry02 (Customized Profile) ==
  Gain{1..3,5} (4 alike) : Gain  Gain=1e6
  Industry02 Power Consumption : FromWorkspace  VariableName=industryphouse02  OutputAfterFinalValue=Holding final value
      mask Display: image('C:\Users\Aryan Ritwajeet Jha\Desktop\CMS Desktop\3-2 2018-19\Mine\EEE F366\Foraged\Images\images.jpg');
  Power transaction with Electric Utility : FromWorkspace  VariableName=industry02  OutputAfterFinalValue=Holding final value
      mask Display: image('C:\Users\Aryan Ritwajeet Jha\Desktop\CMS Desktop\3-2 2018-19\Mine\EEE F366\Foraged\Images\index3.jpg');
  Solar Power : FromWorkspace  VariableName=industrypsolar02  OutputAfterFinalValue=Holding final value
      mask Display: image('C:\Users\Aryan Ritwajeet Jha\Desktop\CMS Desktop\3-2 2018-19\Mine\EEE F366\Foraged\Images\MIT-PPA-1_0.jpg');
  Wind Power : FromWorkspace  VariableName=industrypwind02  OutputAfterFinalValue=Holding final value
      mask Display: image('C:\Users\Aryan Ritwajeet Jha\Desktop\CMS Desktop\3-2 2018-19\Mine\EEE F366\Foraged\Images\index2.jpg');
  Out1 : Outport
  Out2 : Outport  Port=2
  Out3 : Outport  Port=3
  Out4 : Outport  Port=4
  wires:
  Gain3/1 -> Out4/1
  Power transaction with Electric Utility/1 -> Gain3/1
  Wind Power/1 -> Gain2/1
  Solar Power/1 -> Gain1/1
  Gain5/1 -> Out1/1
  Industry02 Power Consumption/1 -> Gain5/1
  Gain1/1 -> Out2/1
  Gain2/1 -> Out3/1

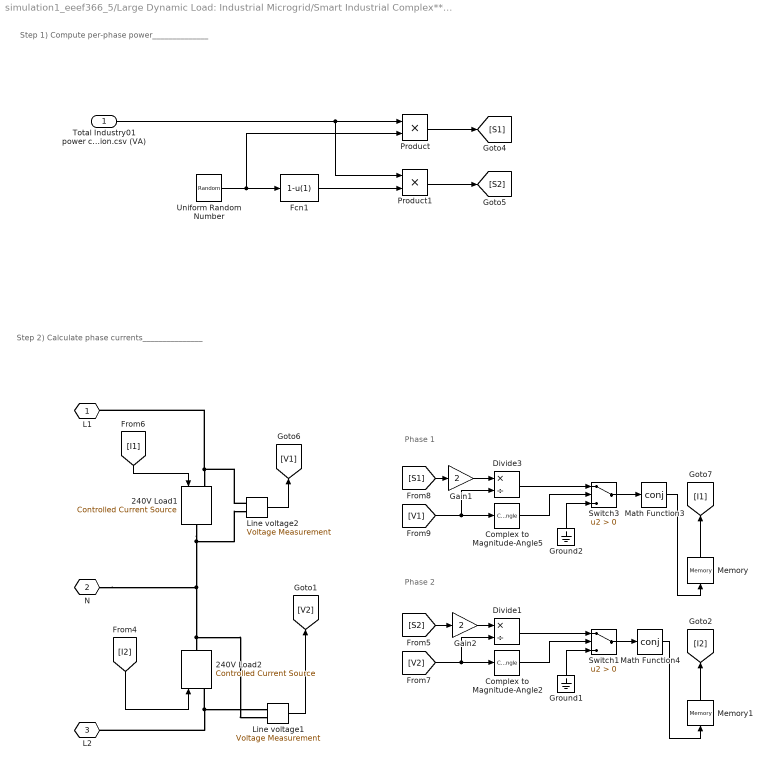
== system simulation1_eeef366_5/Large Dynamic Load: Industrial Microgrid/Smart Industrial Complex**/Industry01 ==
  note: Phase 2
  note: Phase 1
  note: Step 2) Calculate phase currents_______________
  note: Step 1) Compute per-phase power______________
  Total Industry01 power consumption.csv (VA) : Inport
  240V Load1 : powerlib/Electrical Sources/Controlled Current Source  Initialize=off  Source_Type=AC  Amplitude=0  Phase=0  Frequency=0  Measurements=None
  240V Load2 : powerlib/Electrical Sources/Controlled Current Source  Initialize=off  Source_Type=AC  Amplitude=0  Phase=0  Frequency=0  Measurements=None
  Complex to Magnitude-Angle2 : ComplexToMagnitudeAngle  Output=Magnitude
  Complex to Magnitude-Angle5 : ComplexToMagnitudeAngle  Output=Magnitude
  Divide1 : Product  Inputs=*/
  Divide3 : Product  Inputs=*/
  Fcn1 : Fcn  Expr=1-u(1)
  Gain1 : Gain  Gain=2
  Gain2 : Gain  Gain=2
  Ground1 : Ground
  Ground2 : Ground
  Line voltage1 : powerlib/Measurements/Voltage Measurement  Tag=PoWeRsYsTeMmEaSuReMeNt  PhasorSimulation=on  OutputType=Complex  PSBequivalent=0
  Line voltage2 : powerlib/Measurements/Voltage Measurement  Tag=PoWeRsYsTeMmEaSuReMeNt  PhasorSimulation=on  OutputType=Complex  PSBequivalent=0
  Math Function3 : Math  Operator=conj  SaturateOnIntegerOverflow=on
  Math Function4 : Math  Operator=conj  SaturateOnIntegerOverflow=on
  Memory : Memory
  Memory1 : Memory
  Product : Product  RndMeth=Zero
  Product1 : Product  RndMeth=Zero
  Switch1 : Switch  Criteria=u2 > Threshold
  Switch3 : Switch  Criteria=u2 > Threshold
  Uniform Random Number : UniformRandomNumber  Minimum=0
  L1 : PMIOPort  Tag=PMCPort  Port=1  Side=Left
  N : PMIOPort  Tag=PMCPort  Port=2  Side=Left
  L2 : PMIOPort  Tag=PMCPort  Port=3  Side=Left
  wires:
  Total Industry01 power consumption.csv (VA)/1 -> Product/1, Product1/1
  Gain2/1 -> Divide1/1
  Gain1/1 -> Divide3/1
  Math Function4/1 -> Memory1/1
  Math Function3/1 -> Memory/1
  Fcn1/1 -> Product1/2
  Uniform Random Number/1 -> Fcn1/1, Product/2
  [I1] -> 240V Load1/1
  Switch1/1 -> Math Function4/1
  Ground1/1 -> Switch1/3
  Complex to Magnitude-Angle2/1 -> Switch1/2
  Divide1/1 -> Switch1/1
  [V2] -> Complex to Magnitude-Angle2/1, Divide1/2
  [S2] -> Gain2/1
  [I2] -> 240V Load2/1
  Line voltage1/1 -> [V2]
  Switch3/1 -> Math Function3/1
  Ground2/1 -> Switch3/3
  Complex to Magnitude-Angle5/1 -> Switch3/2
  Divide3/1 -> Switch3/1
  [V1] -> Divide3/2, Complex to Magnitude-Angle5/1
  [S1] -> Gain1/1
  Line voltage2/1 -> [V1]
  Product/1 -> [S1]
  Product1/1 -> [S2]
  Memory/1 -> [I1]
  Memory1/1 -> [I2]
  connections:
  L2/RConn1 -- Line voltage1/LConn1 -- 240V Load2/LConn1
  Line voltage2/LConn1 -- L1/RConn1 -- 240V Load1/LConn1
  N/RConn1 -- Line voltage1/LConn2 -- 240V Load2/RConn1 -- 240V Load1/RConn1 -- Line voltage2/LConn2

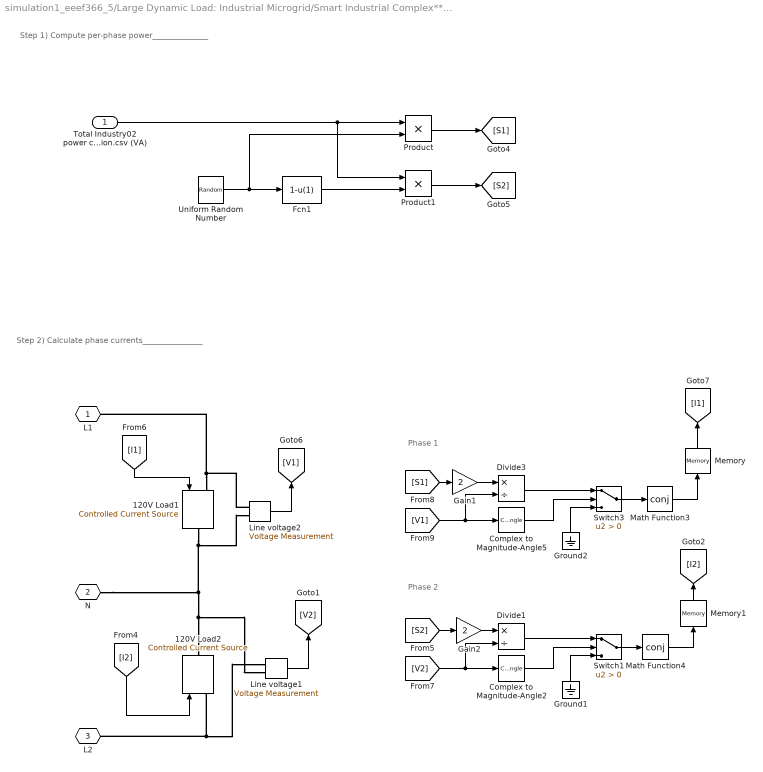
== system simulation1_eeef366_5/Large Dynamic Load: Industrial Microgrid/Smart Industrial Complex**/Industry02 ==
  note: Step 1) Compute per-phase power______________
  note: Step 2) Calculate phase currents_______________
  note: Phase 1
  note: Phase 2
  Total Industry02 power consumption.csv (VA) : Inport
  120V Load1 : powerlib/Electrical Sources/Controlled Current Source  Initialize=off  Source_Type=AC  Amplitude=0  Phase=0  Frequency=0  Measurements=None
  120V Load2 : powerlib/Electrical Sources/Controlled Current Source  Initialize=off  Source_Type=AC  Amplitude=0  Phase=0  Frequency=0  Measurements=None
  Complex to Magnitude-Angle2 : ComplexToMagnitudeAngle  Output=Magnitude
  Complex to Magnitude-Angle5 : ComplexToMagnitudeAngle  Output=Magnitude
  Divide1 : Product  Inputs=*/
  Divide3 : Product  Inputs=*/
  Fcn1 : Fcn  Expr=1-u(1)
  Gain1 : Gain  Gain=2
  Gain2 : Gain  Gain=2
  Ground1 : Ground
  Ground2 : Ground
  Line voltage1 : powerlib/Measurements/Voltage Measurement  Tag=PoWeRsYsTeMmEaSuReMeNt  PhasorSimulation=on  OutputType=Complex  PSBequivalent=0
  Line voltage2 : powerlib/Measurements/Voltage Measurement  Tag=PoWeRsYsTeMmEaSuReMeNt  PhasorSimulation=on  OutputType=Complex  PSBequivalent=0
  Math Function3 : Math  Operator=conj  SaturateOnIntegerOverflow=on
  Math Function4 : Math  Operator=conj  SaturateOnIntegerOverflow=on
  Memory : Memory
  Memory1 : Memory
  Product : Product  RndMeth=Zero
  Product1 : Product  RndMeth=Zero
  Switch1 : Switch  Criteria=u2 > Threshold
  Switch3 : Switch  Criteria=u2 > Threshold
  Uniform Random Number : UniformRandomNumber  Minimum=0
  L1 : PMIOPort  Tag=PMCPort  Port=1  Side=Left
  N : PMIOPort  Tag=PMCPort  Port=2  Side=Left
  L2 : PMIOPort  Tag=PMCPort  Port=3  Side=Left
  wires:
  Memory1/1 -> [I2]
  Memory/1 -> [I1]
  Product1/1 -> [S2]
  Product/1 -> [S1]
  Line voltage2/1 -> [V1]
  [S1] -> Gain1/1
  [V1] -> Complex to Magnitude-Angle5/1, Divide3/2
  Divide3/1 -> Switch3/1
  Complex to Magnitude-Angle5/1 -> Switch3/2
  Ground2/1 -> Switch3/3
  Switch3/1 -> Math Function3/1
  Line voltage1/1 -> [V2]
  [I2] -> 120V Load2/1
  [S2] -> Gain2/1
  [V2] -> Divide1/2, Complex to Magnitude-Angle2/1
  Divide1/1 -> Switch1/1
  Complex to Magnitude-Angle2/1 -> Switch1/2
  Ground1/1 -> Switch1/3
  Switch1/1 -> Math Function4/1
  [I1] -> 120V Load1/1
  Uniform Random Number/1 -> Product/2, Fcn1/1
  Fcn1/1 -> Product1/2
  Math Function3/1 -> Memory/1
  Math Function4/1 -> Memory1/1
  Gain1/1 -> Divide3/1
  Gain2/1 -> Divide1/1
  Total Industry02 power consumption.csv (VA)/1 -> Product1/1, Product/1
  connections:
  120V Load1/LConn1 -- L1/RConn1 -- Line voltage2/LConn1
  120V Load2/LConn1 -- Line voltage1/LConn1 -- L2/RConn1
  N/RConn1 -- 120V Load1/RConn1 -- Line voltage2/LConn2 -- 120V Load2/RConn1 -- Line voltage1/LConn2

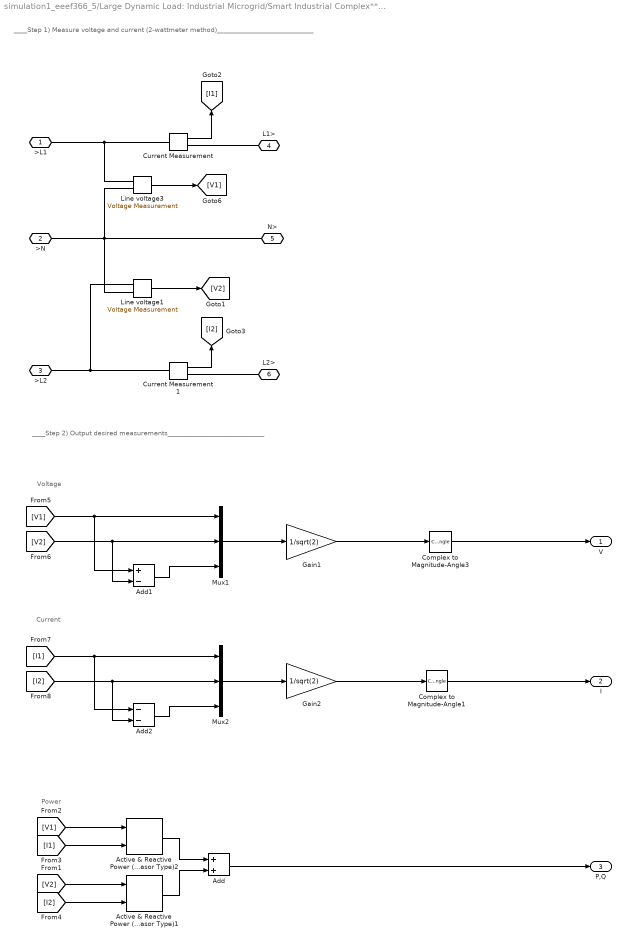
== system simulation1_eeef366_5/Large Dynamic Load: Industrial Microgrid/Smart Industrial Complex**/Smart Meter Industry01 ==
  note: ____Step 1) Measure voltage and current (2-wattmeter method)_____________________________
  note: ____Step 2) Output desired measurements_____________________________
  note: Power
  note: Current
  note: Voltage
  Active & Reactive Power (Phasor Type)1 : powerlib_extras/Phasor Library/Active & Reactive Power (Phasor Type)
  Active & Reactive Power (Phasor Type)2 : powerlib_extras/Phasor Library/Active & Reactive Power (Phasor Type)
  Add : Sum
  Add1 : Sum  Inputs=+-
  Add2 : Sum  Inputs=--
  Complex to Magnitude-Angle1 : ComplexToMagnitudeAngle  Output=Magnitude
  Complex to Magnitude-Angle3 : ComplexToMagnitudeAngle  Output=Magnitude
  Current Measurement : powerlib/Measurements/Current Measurement  PhasorSimulation=on  OutputType=Complex  PSBequivalent=0
  Current Measurement1 : powerlib/Measurements/Current Measurement  PhasorSimulation=on  OutputType=Complex  PSBequivalent=0
  Gain1 : Gain  Gain=1/sqrt(2)
  Gain2 : Gain  Gain=1/sqrt(2)
  Line voltage1 : powerlib/Measurements/Voltage Measurement  Tag=PoWeRsYsTeMmEaSuReMeNt  PhasorSimulation=on  OutputType=Complex  PSBequivalent=0
  Line voltage3 : powerlib/Measurements/Voltage Measurement  Tag=PoWeRsYsTeMmEaSuReMeNt  PhasorSimulation=on  OutputType=Complex  PSBequivalent=0
  Mux1 : Mux  Inputs=3
  Mux2 : Mux  Inputs=3
  >L1 : PMIOPort  Port=1  Side=Left
      settings: AttributesFormatString=%<Side>
  >N : PMIOPort  Port=2  Side=Left
      settings: AttributesFormatString=%<Side>
  >L2 : PMIOPort  Port=3  Side=Left
      settings: AttributesFormatString=%<Side>
  L1> : PMIOPort  Port=4  Side=Right
      settings: AttributesFormatString=%<Side>
  N> : PMIOPort  Port=5  Side=Right
      settings: AttributesFormatString=%<Side>
  L2> : PMIOPort  Port=6  Side=Right
      settings: AttributesFormatString=%<Side>
  V : Outport
  I : Outport  Port=2
  P,Q : Outport  Port=3
  wires:
  Line voltage3/1 -> [V1]
  Line voltage1/1 -> [V2]
  Current Measurement/1 -> [I1]
  Current Measurement1/1 -> [I2]
  [V1] -> Active & Reactive Power (Phasor Type)2/1
  [I1] -> Active & Reactive Power (Phasor Type)2/2
  [V2] -> Active & Reactive Power (Phasor Type)1/1
  [I2] -> Active & Reactive Power (Phasor Type)1/2
  Active & Reactive Power (Phasor Type)2/1 -> Add/1
  Active & Reactive Power (Phasor Type)1/1 -> Add/2
  Add/1 -> P,Q/1
  [V1] -> Mux1/1, Add1/1
  [V2] -> Mux1/2, Add1/2
  Add1/1 -> Mux1/3
  Mux1/1 -> Gain1/1
  [I1] -> Add2/1, Mux2/1
  [I2] -> Add2/2, Mux2/2
  Add2/1 -> Mux2/3
  Mux2/1 -> Gain2/1
  Gain1/1 -> Complex to Magnitude-Angle3/1
  Gain2/1 -> Complex to Magnitude-Angle1/1
  Complex to Magnitude-Angle3/1 -> V/1
  Complex to Magnitude-Angle1/1 -> I/1
  connections:
  >L1/RConn1 -- Current Measurement/LConn1 -- Line voltage3/LConn1
  Current Measurement/RConn1 -- L1>/RConn1
  N>/RConn1 -- Line voltage3/LConn2 -- Line voltage1/LConn2 -- >N/RConn1
  >L2/RConn1 -- Line voltage1/LConn1 -- Current Measurement1/LConn1
  L2>/RConn1 -- Current Measurement1/RConn1

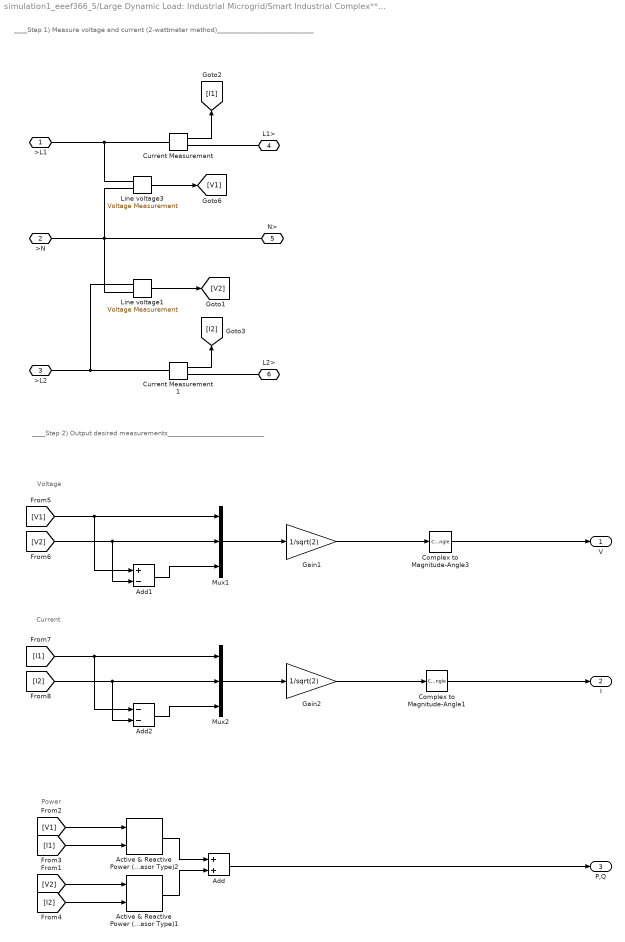
== system simulation1_eeef366_5/Large Dynamic Load: Industrial Microgrid/Smart Industrial Complex**/Smart Meter Industry02 ==
  note: Voltage
  note: Current
  note: Power
  note: ____Step 2) Output desired measurements_____________________________
  note: ____Step 1) Measure voltage and current (2-wattmeter method)_____________________________
  Active & Reactive Power (Phasor Type)1 : powerlib_extras/Phasor Library/Active & Reactive Power (Phasor Type)
  Active & Reactive Power (Phasor Type)2 : powerlib_extras/Phasor Library/Active & Reactive Power (Phasor Type)
  Add : Sum
  Add1 : Sum  Inputs=+-
  Add2 : Sum  Inputs=--
  Complex to Magnitude-Angle1 : ComplexToMagnitudeAngle  Output=Magnitude
  Complex to Magnitude-Angle3 : ComplexToMagnitudeAngle  Output=Magnitude
  Current Measurement : powerlib/Measurements/Current Measurement  PhasorSimulation=on  OutputType=Complex  PSBequivalent=0
  Current Measurement1 : powerlib/Measurements/Current Measurement  PhasorSimulation=on  OutputType=Complex  PSBequivalent=0
  Gain1 : Gain  Gain=1/sqrt(2)
  Gain2 : Gain  Gain=1/sqrt(2)
  Line voltage1 : powerlib/Measurements/Voltage Measurement  Tag=PoWeRsYsTeMmEaSuReMeNt  PhasorSimulation=on  OutputType=Complex  PSBequivalent=0
  Line voltage3 : powerlib/Measurements/Voltage Measurement  Tag=PoWeRsYsTeMmEaSuReMeNt  PhasorSimulation=on  OutputType=Complex  PSBequivalent=0
  Mux1 : Mux  Inputs=3
  Mux2 : Mux  Inputs=3
  >L1 : PMIOPort  Port=1  Side=Left
      settings: AttributesFormatString=%<Side>
  >N : PMIOPort  Port=2  Side=Left
      settings: AttributesFormatString=%<Side>
  >L2 : PMIOPort  Port=3  Side=Left
      settings: AttributesFormatString=%<Side>
  L1> : PMIOPort  Port=4  Side=Right
      settings: AttributesFormatString=%<Side>
  N> : PMIOPort  Port=5  Side=Right
      settings: AttributesFormatString=%<Side>
  L2> : PMIOPort  Port=6  Side=Right
      settings: AttributesFormatString=%<Side>
  V : Outport
  I : Outport  Port=2
  P,Q : Outport  Port=3
  wires:
  Complex to Magnitude-Angle1/1 -> I/1
  Complex to Magnitude-Angle3/1 -> V/1
  Gain2/1 -> Complex to Magnitude-Angle1/1
  Gain1/1 -> Complex to Magnitude-Angle3/1
  Mux2/1 -> Gain2/1
  Add2/1 -> Mux2/3
  [I2] -> Mux2/2, Add2/2
  [I1] -> Mux2/1, Add2/1
  Mux1/1 -> Gain1/1
  Add1/1 -> Mux1/3
  [V2] -> Add1/2, Mux1/2
  [V1] -> Add1/1, Mux1/1
  Add/1 -> P,Q/1
  Active & Reactive Power (Phasor Type)1/1 -> Add/2
  Active & Reactive Power (Phasor Type)2/1 -> Add/1
  [I2] -> Active & Reactive Power (Phasor Type)1/2
  [V2] -> Active & Reactive Power (Phasor Type)1/1
  [I1] -> Active & Reactive Power (Phasor Type)2/2
  [V1] -> Active & Reactive Power (Phasor Type)2/1
  Current Measurement1/1 -> [I2]
  Current Measurement/1 -> [I1]
  Line voltage1/1 -> [V2]
  Line voltage3/1 -> [V1]
  connections:
  L2>/RConn1 -- Current Measurement1/RConn1
  Line voltage1/LConn1 -- >L2/RConn1 -- Current Measurement1/LConn1
  Line voltage3/LConn2 -- N>/RConn1 -- >N/RConn1 -- Line voltage1/LConn2
  Current Measurement/RConn1 -- L1>/RConn1
  Current Measurement/LConn1 -- >L1/RConn1 -- Line voltage3/LConn1
